simulink model "provaArduinoWithServo"  (R2016b)
settings: Solver=ode3  StartTime=0.0  StopTime=10.0  RelTol=1e-3  EnableMultiTasking=on
undefined symbols (not defined in the file): sigbuilder_block
libraries: arduinolib x6
settings Model: SimulationMode=external  ExtModeTrigDuration=2  Creator=user  LastModifiedBy=toni
settings DataIOCC: LimitDataPoints=on  SaveFormat=Array
settings OptimizationCC: MaxStackSize=64
settings DebuggingCC: UnderspecifiedInitializationDetection=Classic  MergeDetectMultiDrivingBlocksExec=none  ParameterTunabilityLossMsg=error  StateNameClashWarn=warning  SFUnexpectedBacktrackingDiag=warning  SFNoUnconditionalDefaultTransitionDiag=warning  SFExecutionAtInitializationDiag=none
settings HardwareCC: ProdBitPerInt=16  ProdBitPerPointer=16  ProdBitPerSizeT=16  ProdBitPerPtrDiffT=16  ProdLargestAtomicFloat=None  ProdWordSize=8  ProdHWDeviceType=Atmel->AVR
settings ModelReferenceCC: PropagateSignalLabelsOutOfModel=off
settings SFSimCC: SimBuildMode=sf_nonincremental_build
settings RTWCC: SystemTargetFile=ert.tlc  HardwareBoard=Arduino Uno  TLCOptions=-aInlineSetEventsForThisBaseRateFcn=TLC_FALSE -aSuppressMultiTaskScheduler=TLC_FALSE -aRateBasedStepFcn=1  TemplateMakefile=ert_default_tmf  Description=Embedded Coder  GenerateReport=on  RTWVerbose=off  Toolchain=Arduino AVR v1.6.7  BuildConfiguration=Faster Runs  IncludeHyperlinkInReport=on  LaunchReport=on  GenerateTraceInfo=on  GenerateTraceReport=on  GenerateTraceReportSl=on  GenerateTraceReportSf=on  GenerateTraceReportEml=on
settings CodeAppCC: ForceParamTrailComments=on  IgnoreCustomStorageClasses=off  OperatorAnnotations=on  SimulinkDataObjDesc=on  SFDataObjDesc=on  MATLABFcnDesc=on  InsertBlockDesc=on  MATLABSourceComments=on
settings ERTTargetCC: SupportContinuousTime=on  SupportVariableSizeSignals=on
settings ConfigComp: CovMetricSettings=dw  CovHtmlReporting=on  CovSaveCumulativeToWorkspaceVar=on  CovSaveSingleToWorkspaceVar=on  CovExternalEMLEnable=off

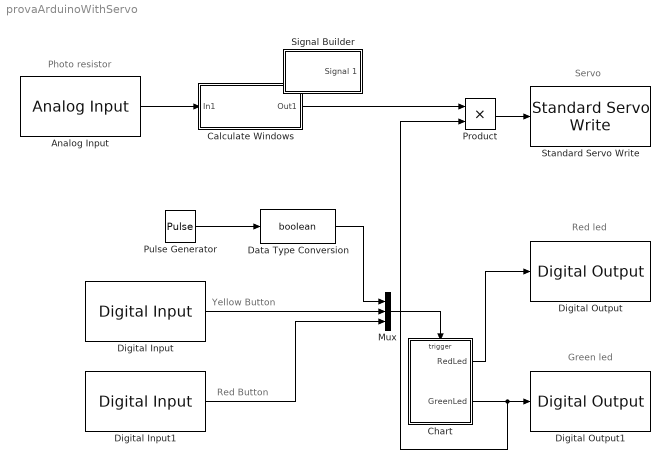
== system provaArduinoWithServo ==
  note: Green led
  note: Red led
  note: Servo
  note: Photo resistor
  note: Red Button
  note: Yellow Button
  Analog Input : arduinolib/Analog Input  pinNumber=4  sampleTime=0.1  blockPlatform=arduino
  Calculate Windows : Subsystem
  Chart : Stateflow chart  TreatAsAtomicUnit=on
  Data Type Conversion : DataTypeConversion  OutDataTypeStr=boolean
  Digital Input : arduinolib/Digital Input  pinNumber=7  sampleTime=0.1  blockPlatform=arduino
  Digital Input1 : arduinolib/Digital Input  pinNumber=6  sampleTime=0.1  blockPlatform=arduino
  Digital Output : arduinolib/Digital Output  pinNumber=9  blockPlatform=arduino
  Digital Output1 : arduinolib/Digital Output  pinNumber=8  blockPlatform=arduino
  Mux : Mux  Inputs=3
  Product : Product  OutDataTypeStr=uint8
  Pulse Generator : DiscretePulseGenerator  Period=10  PulseWidth=5  SampleTime=0.1
  Standard Servo Write : arduinolib/Standard Servo Write  pinNumber=10  blockPlatform=arduino
  Signal Builder : Subsystem  Tag=STV Subsys  IOType=siggen  LoadFcn=sigbuilder_block('load');  StartFcn=sigbuilder_block('start');  StopFcn=sigbuilder_block('stop');  ClipboardFcn=sigbuilder_block('clipboard');  mask(Sigbuilder block){tuvar=[0:10]}
      mask help: Sigbuilder GUI
      mask init:
      | if ~strcmp(get_param(bdroot(gcbh),'SimulationStatus'),'stopped') tuvar = sigbuilder_block('maskInit'); end
      settings: CopyFcn=sigbuilder_block('copy');  DeleteFcn=sigbuilder_block('delete');  ModelCloseFcn=sigbuilder_block('modelClose');  PreSaveFcn=sigbuilder_block('preSave');  PauseFcn=sigbuilder_block('pause');  ContinueFcn=sigbuilder_block('continue');  NameChangeFcn=sigbuilder_block('namechange');  OpenFcn=sigbuilder_block('open',[437.6 199.2 550.4 400 ]);  CloseFcn=sigbuilder_block('close');
      mask Display: plot(0, 0, 100, 100,[2, 2, 32, 32, 2], [68, 8, 8, 68, 68],[32, 2], [38, 38], [32, 19, 2],[53, 60, 44], [32, 17, 17, 2],[16, 16, 31, 31]);txt = getActiveGroup(gcbh);text(2, 100, txt,'verticalAlignment', 'top');
  wires:
  Chart/1(RedLed) -> Digital Output/1
  Chart/2(GreenLed) -> Product/2, Digital Output1/1
  Digital Input/1 -> Mux/2
  Pulse Generator/1 -> Data Type Conversion/1
  Data Type Conversion/1 -> Mux/1
  Mux/1 -> Chart/Trigger
  Digital Input1/1 -> Mux/3
  Product/1 -> Standard Servo Write/1
  Analog Input/1 -> Calculate Windows/1(In1)
  Calculate Windows/1(Out1) -> Product/1

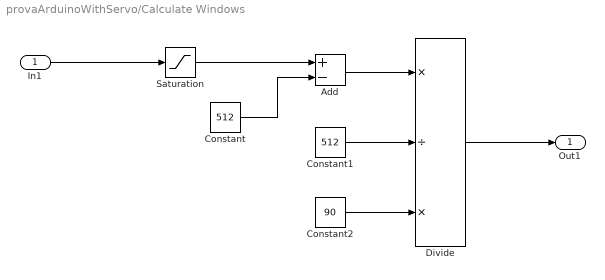
== system provaArduinoWithServo/Calculate Windows ==
  In1 : Inport
  Add : Sum  Inputs=+-
  Constant : Constant  Value=512
  Constant1 : Constant  Value=512
  Constant2 : Constant  Value=90
  Divide : Product  Inputs=*/*
  Saturation : Saturate  UpperLimit=1023  LowerLimit=512  OutDataTypeStr=Inherit: Inherit via back propagation
  Out1 : Outport
  wires:
  In1/1 -> Saturation/1
  Saturation/1 -> Add/1
  Constant/1 -> Add/2
  Add/1 -> Divide/1
  Constant1/1 -> Divide/2
  Constant2/1 -> Divide/3
  Divide/1 -> Out1/1

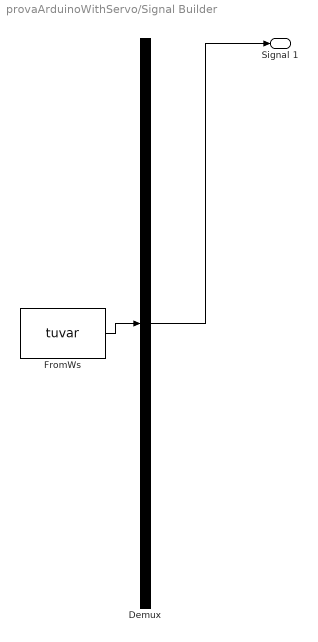
== system provaArduinoWithServo/Signal Builder ==
  Demux : Demux  Tag=STV Demux  Outputs=1
  FromWs : FromWorkspace  Tag=STV FromWs  VariableName=tuvar  SampleTime=0
      SigBuilderData=|
      | common.afterFinalStr = 'Extrapolate'
      | common.sampleTime = 0
      | dataSet.timeRange = [0 10]
      | dataSet.name = 'Group 1'
      | sbobj.Groups.Name = 'Group 1'
      | sbobj.Groups.Signals.Name = 'Signal 1'
      | sbobj.Groups.Signals.XData = [0 4 4 6 6 10]
      | sbobj.Groups.Signals.YData = [0 0 1 1 0 0]
  Signal 1 : Outport  Tag=STV Outport
  wires:
  FromWs/1 -> Demux/1
  Demux/1 -> Signal 1/1

== stateflow chart provaArduinoWithServo/Chart ==
  state main
    state uno [parallel]
      settings: executionOrder=2
      (history)
      state init
      state body
      (default) -> init
      init -> body : click/send(ON,due);
      body -> init : click/send(OFF,due);
    state due [parallel]
      settings: executionOrder=1
      (history)
      state A
        entry:
        RedLed=1;
      state B
        entry:
        RedLed=0;
      A -> A [order 2] : YellowButton/send(GreenON,tre);
      A -> B [order 1] : OFF
      B -> A [order 1] : ON
      B -> B [order 2] : YellowButton/send(GreenOFF,tre);
      (default) -> B
    state tre [parallel]
      settings: executionOrder=3
      (history)
      state C
        entry:
        GreenLed=1;
      state D
        entry:
        GreenLed=0;
      D -> C : GreenON
      C -> D : GreenOFF
      (default) -> D
  state Suspend
    entry:
    RedLed=0;
    GreenLed=0;
  (default) -> main
  Suspend -> main : RedButton
  main -> Suspend : RedButton
  data: RedLed output boolean; GreenLed output boolean
  events: click input RISING_EDGE_EVENT; ON local RISING_EDGE_EVENT; OFF local RISING_EDGE_EVENT; YellowButton input RISING_EDGE_EVENT; RedButton input RISING_EDGE_EVENT; GreenON local FUNCTION_CALL_EVENT; GreenOFF local FUNCTION_CALL_EVENT
